simulink model "lab3_sim"  (R2020b)
settings: Solver=VariableStepAuto  StartTime=0.0  StopTime=100  RelTol=1e-3
values from neighbouring files (symbols this model uses):
  a1 = -1.655    [lab5.m]
  b = 0.385    [lab5.m]
  J = 0.71*10^-3    (= 0.00071)    [lab4.m]
  ke = 0.33    [lab4.m]
  km = 0.33    [lab4.m]
  kp = 35    [lab4.m]
  La = 14.28*10^-3    (= 0.01428)    [lab4.m]
  Ra = 4.2    [lab4.m]
undefined symbols (not defined in the file or in its folder): a2, alpha, c, delta, fmax, g, kem, Psi, Ti
settings Model: Creator=student  LastModifiedBy=student

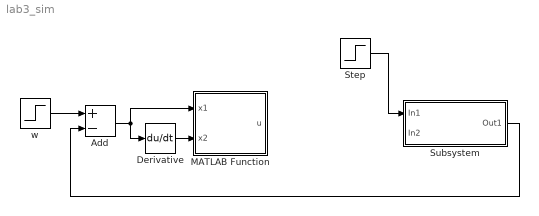
== system lab3_sim ==
  Add : Sum  Inputs=+-
  Derivative : Derivative
  MATLAB Function : MATLAB Function  TreatAsAtomicUnit=on
  Step : Step  Time=0.6  After=-12  SampleTime=0
  Subsystem : Subsystem
  w : Step  SampleTime=0
  wires:
  Step/1 -> Subsystem/1(In1)
  Subsystem/1(Out1) -> Add/2
  w/1 -> Add/1
  Add/1 -> Derivative/1, MATLAB Function/1(x1)
  Derivative/1 -> MATLAB Function/2(x2)

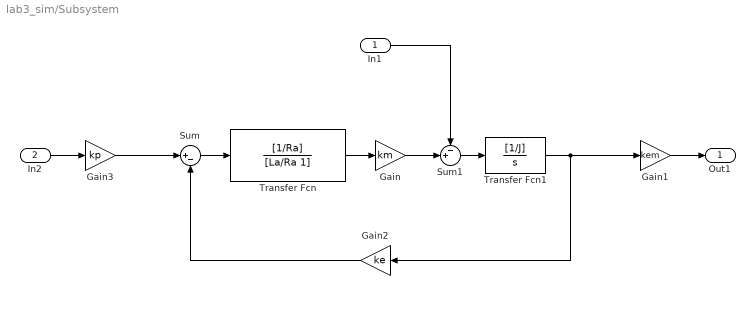
== system lab3_sim/Subsystem ==
  In1 : Inport
  In2 : Inport  Port=2
  Gain : Gain  Gain=km
  Gain1 : Gain  Gain=kem
  Gain2 : Gain  Gain=ke
  Gain3 : Gain  Gain=kp
  Sum : Sum  Inputs=|+-
  Sum1 : Sum  Inputs=-+|
  Transfer Fcn : TransferFcn  Numerator=[1/Ra]  Denominator=[La/Ra 1]
  Transfer Fcn1 : TransferFcn  Numerator=[1/J]  Denominator=[1 0]
  Out1 : Outport
  wires:
  Sum1/1 -> Transfer Fcn1/1
  Sum/1 -> Transfer Fcn/1
  Gain2/1 -> Sum/2
  Gain3/1 -> Sum/1
  Transfer Fcn/1 -> Gain/1
  Transfer Fcn1/1 -> Gain2/1, Gain1/1
  Gain/1 -> Sum1/2
  Gain1/1 -> Out1/1
  In1/1 -> Sum1/1
  In2/1 -> Gain3/1

== matlab function lab3_sim/MATLAB Function ==
  data: x1 input; x2 input; u output; Psi parameter; alpha parameter; g parameter; Ti parameter; c parameter; a1 parameter; a2 parameter; b parameter; fmax parameter; delta parameter
function u = fcn(x1,x2,Psi, alpha, g, Ti, c, a1, a2, b, fmax, delta)
g = c*x1+x2;
alpha=(mod((c^2 - a2*c + a1)*x1)+fmax)/mod(b)*(mod(x1)+1/Ti*())+delta;
